simulink model "CH3_1B"  (R2021b)
settings: Solver=ode45  StartTime=0.0  StopTime=47*20  RelTol=1e-3  EnableMultiTasking=on
settings Model: Creator=my2  LastModifiedBy=82102
settings SolverCC: AlgebraicLoopSolver=TrustRegion
settings DataIOCC: LimitDataPoints=on  SaveFormat=Array  SignalLoggingSaveFormat=ModelDataLogs  ReturnWorkspaceOutputs=off
settings OptimizationCC: LifeSpan=inf
settings DebuggingCC: SolverPrmCheckMsg=warning  MultiTaskDSMMsg=warning  MultiTaskCondExecSysMsg=none  FcnCallInpInsideContextMsg=warning  SFUnexpectedBacktrackingDiag=warning  SFNoUnconditionalDefaultTransitionDiag=warning  SFExecutionAtInitializationDiag=none  SFMachineParentedDataDiag=warning  ArithmeticOperatorsInVariantConditions=warning
settings HardwareCC: ProdBitPerPointer=32  ProdBitPerSizeT=32  ProdBitPerPtrDiffT=32  ProdLargestAtomicFloat=None  ProdIntDivRoundTo=Undefined  ProdEndianess=Unspecified  ProdWordSize=32  ProdHWDeviceType=32-bit Generic
settings ModelReferenceCC: PropagateSignalLabelsOutOfModel=off
settings SFSimCC: SimUseLocalCustomCode=off  CustomCodeUndefinedFunction=UseInterfaceOnly
settings RTWCC: RTWUseLocalCustomCode=off
settings CodeAppCC: StateflowObjectComments=on
settings GRTTargetCC: TargetLangStandard=C89/C90 (ANSI)  CombineOutputUpdateFcns=off  GRTInterface=on
settings ConfigComp: CovMetricSettings=dw  CovSaveCumulativeToWorkspaceVar=on  CovSaveSingleToWorkspaceVar=on  CovExternalEMLEnable=off

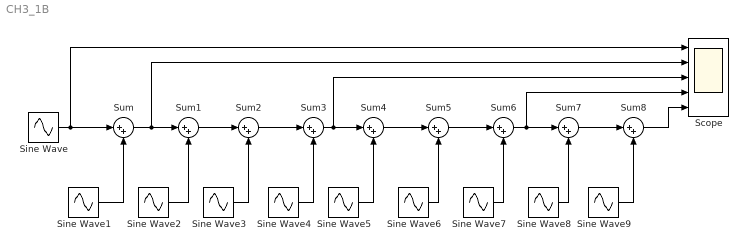
== system CH3_1B ==
  Scope : Scope  NumInputPorts=5
  Sine Wave : Sin  Amplitude=4/pi  Frequency=2*pi/25  Phase=pi/2  SampleTime=0.1
  Sine Wave1 : Sin  Amplitude=4/pi*(-1/3)  Frequency=3*2*pi/25  Phase=pi/2  SampleTime=0.1
  Sine Wave2 : Sin  Amplitude=4/pi*(1/5)  Frequency=5*2*pi/25  Phase=pi/2  SampleTime=0.1
  Sine Wave3 : Sin  Amplitude=4/pi *(-1/7)  Frequency=7*2*pi/25  Phase=pi/2  SampleTime=0.1
  Sine Wave4 : Sin  Amplitude=2*pi/25 *(1/9)  Frequency=4/pi *9  Phase=pi/2  SampleTime=0.1
  Sine Wave5 : Sin  Amplitude=2*pi/25*(-1/11)  Frequency=11*4/pi  Phase=pi/2  SampleTime=0.1
  Sine Wave6 : Sin  Amplitude=2*pi/25*(1/13)  Frequency=13*4/pi  Phase=pi/2  SampleTime=0.1
  Sine Wave7 : Sin  Amplitude=2*pi/25*(-1/15)  Frequency=15*4/pi  Phase=pi/2  SampleTime=0.1
  Sine Wave8 : Sin  Amplitude=2*pi/25*(1/17)  Frequency=17*4/pi  Phase=pi/2  SampleTime=0.1
  Sine Wave9 : Sin  Amplitude=2*pi/25*(-1/19)  Frequency=19*4/pi  Phase=pi/2  SampleTime=0.1
  Sum{,1..8} (9 alike) : Sum  Inputs=|++
  wires:
  Sine Wave/1 -> Scope/1, Sum/1
  Sine Wave1/1 -> Sum/2
  Sum/1 -> Scope/2, Sum1/1
  Sine Wave2/1 -> Sum1/2
  Sum1/1 -> Sum2/1
  Sum2/1 -> Sum3/1
  Sum3/1 -> Scope/3, Sum4/1
  Sum4/1 -> Sum5/1
  Sum5/1 -> Sum6/1
  Sum6/1 -> Scope/4, Sum7/1
  Sine Wave3/1 -> Sum2/2
  Sine Wave4/1 -> Sum3/2
  Sine Wave5/1 -> Sum4/2
  Sine Wave6/1 -> Sum5/2
  Sine Wave7/1 -> Sum6/2
  Sine Wave8/1 -> Sum7/2
  Sine Wave9/1 -> Sum8/2
  Sum7/1 -> Sum8/1
  Sum8/1 -> Scope/5
